simulink model "Lab3_CAES"  (R2020a)
settings: Solver=VariableStepAuto  StartTime=0.0  StopTime=1500  RelTol=1e-3
settings Model: Creator=mitch  LastModifiedBy=mitch

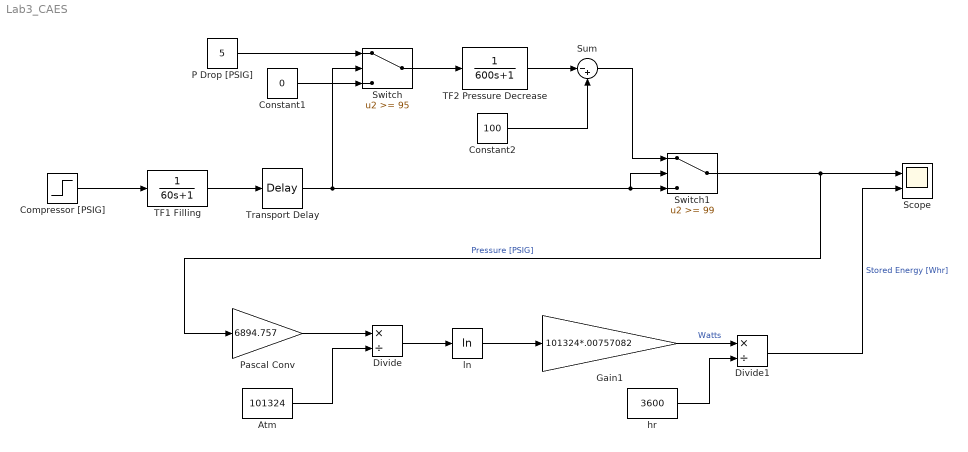
== system Lab3_CAES ==
  Atm : Constant  Value=101324
  Compressor [PSIG] : Step  After=100  SampleTime=0
  Constant1 : Constant  Value=0
  Constant2 : Constant  Value=100
  Divide : Product  Inputs=*/
  Divide1 : Product  Inputs=*/
  Gain1 : Gain  Gain=101324*.00757082
  P Drop [PSIG] : Constant  Value=5
  Pascal Conv : Gain  Gain=6894.757
  Scope : Scope  NumInputPorts=2
  Sum : Sum  Inputs=|-+
  Switch : Switch  Threshold=95
  Switch1 : Switch  Threshold=99
  TF1 Filling : TransferFcn  Denominator=[60 1]
  TF2 Pressure Decrease : TransferFcn  Denominator=[600 1]
  Transport Delay : TransportDelay
  hr : Constant  Value=3600
  ln : Math  Operator=log  SaturateOnIntegerOverflow=on
  wires:
  Compressor [PSIG]/1 -> TF1 Filling/1
  Constant2/1 -> Sum/2
  TF2 Pressure Decrease/1 -> Sum/1
  Pascal Conv/1 -> Divide/1
  Atm/1 -> Divide/2
  Divide/1 -> ln/1
  ln/1 -> Gain1/1
  Gain1/1 -> Divide1/1  "Watts"
  hr/1 -> Divide1/2
  Divide1/1 -> Scope/2  "Stored Energy [Whr]"
  TF1 Filling/1 -> Transport Delay/1
  P Drop [PSIG]/1 -> Switch/1
  Transport Delay/1 -> Switch/2, Switch1/2, Switch1/3
  Constant1/1 -> Switch/3
  Switch/1 -> TF2 Pressure Decrease/1
  Sum/1 -> Switch1/1
  Switch1/1 -> Pascal Conv/1, Scope/1  "Pressure [PSIG]"
